simulink model "simulunk4"  (R2016a)
settings: Solver=VariableStepAuto  StartTime=0.0  StopTime=10.0  RelTol=1e-3
undefined symbols (not defined in the file): a, b
settings Model: Creator=user  LastModifiedBy=user

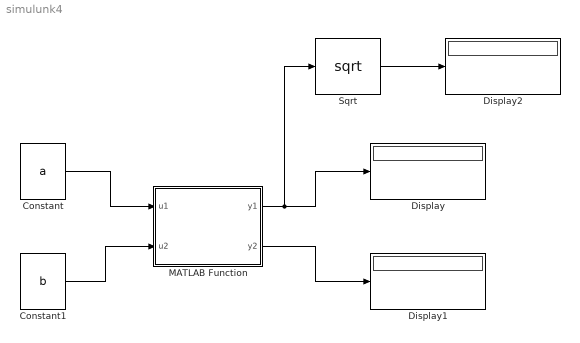
== system simulunk4 ==
  Constant : Constant  Value=a
  Constant1 : Constant  Value=b
  Display : Display
  Display1 : Display
  Display2 : Display
  MATLAB Function : MATLAB Function  TreatAsAtomicUnit=on
  Sqrt : Sqrt  SaturateOnIntegerOverflow=on
  wires:
  Constant/1 -> MATLAB Function/1(u1)
  MATLAB Function/1(y1) -> Sqrt/1, Display/1
  Constant1/1 -> MATLAB Function/2(u2)
  MATLAB Function/2(y2) -> Display1/1
  Sqrt/1 -> Display2/1

== matlab function simulunk4/MATLAB Function ==
  data: u1 input; y1 output; u2 input; y2 output
function [y1,y2] = fcn(u1,u2)
%#codegen
if u1>u2
    y1=u1+u2;
    y2=u1-u2;
else
    y1=u1*u2;
    y2=u1/u2;
end
